simulink model "PID_noise_filter"  (R2020b)
settings: Solver=VariableStepAuto  StartTime=0.0  StopTime=300  RelTol=1e-3
libraries: pid_lib x6, simulink x4, dsparch4 x2
settings Model: Creator=Obsidian  LastModifiedBy=Obsidian

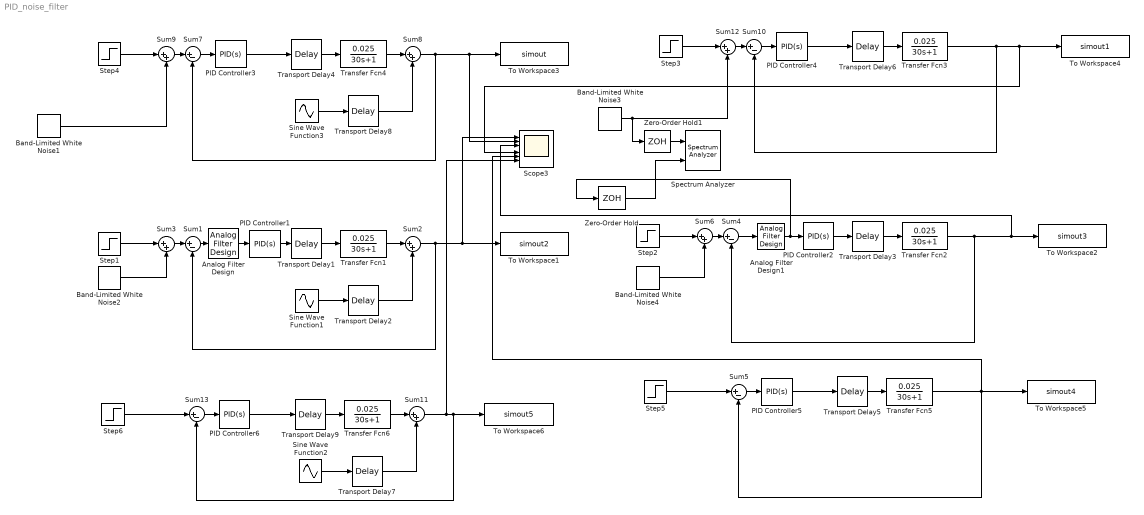
== system PID_noise_filter ==
  Analog Filter Design : dsparch4/Analog Filter Design  method=Butterworth  filttype=Lowpass  N=5  Wlo=62.8  Whi=80  Rp=2  Rs=40
  Analog Filter Design1 : dsparch4/Analog Filter Design  method=Butterworth  filttype=Lowpass  N=5  Wlo=62.8  Whi=80  Rp=2  Rs=40
  Band-Limited White Noise{1..4} (4 alike) : simulink/Sources/Band-Limited White Noise  Cov=[0.1]  Ts=0.01  seed=[23341]
  PID Controller{1..6} (6 alike) : pid_lib/PID Controller  Controller=PID  Form=Parallel  TimeDomain=Continuous-time  UseExternalTs=off  SampleTime=-1  IntegratorMethod=Forward Euler  FilterMethod=Forward Euler  ControllerParametersSource=internal  P=91.1934989789184  I=4.3602787236588  D=159.272174237234  UseFilter=on  N=0.14098946944392  TunerSelectOption=Transfer Function Based (PID Tuner App)  InitialConditionSource=internal  InitialConditionForIntegrator=0  InitialConditionForFilter=0  DifferentiatorICPrevScaledInput=0  ExternalReset=none  TrackingMode=off  Kt=1  LimitOutput=on  SatLimitsSource=internal  UpperSaturationLimit=200  LowerSaturationLimit=0  LinearizeAsGain=on  AntiWindupMode=none  Kb=1  POutMin=[]  POutMax=[]  IOutMin=[]  IOutMax=[]  DOutMin=[]  DOutMax=[]  NOutMin=[]  NOutMax=[]  SumOutMin=[]  SumOutMax=[]  SaturationOutMin=[]  SaturationOutMax=[]  PParamMin=[]  PParamMax=[]  IParamMin=[]  IParamMax=[]  DParamMin=[]  DParamMax=[]  NParamMin=[]  NParamMax=[]  KbParamMin=[]  KbParamMax=[]  KtParamMin=[]  KtParamMax=[]  KbOutMin=[]  KbOutMax=[]  KtOutMin=[]  KtOutMax=[]  IntegratorOutMin=[]  IntegratorOutMax=[]  FilterOutMin=[]  FilterOutMax=[]  SumI1OutMin=[]  SumI1OutMax=[]  SumI2OutMin=[]  SumI2OutMax=[]  SumI3OutMin=[]  SumI3OutMax=[]  SumI4OutMin=[]  SumI4OutMax=[]  SumDOutMin=[]  SumDOutMax=[]  DifferentiatorOutMin=[]  DifferentiatorOutMax=[]  FilterDiffOutCoefMin=[]  FilterDiffOutCoefMax=[]  ReciprocalOutMin=[]  ReciprocalOutMax=[]  SumDenOutMin=[]  SumDenOutMax=[]  SumNumOutMin=[]  SumNumOutMax=[]  DivideOutMin=[]  DivideOutMax=[]  UdiffTsProdOutMin=[]  UdiffTsProdOutMax=[]  NTsProdOutMin=[]  NTsProdOutMax=[]  UintegralTsProdOutMin=[]  UintegralTsProdOutMax=[]  UngainTsProdOutMin=[]  UngainTsProdOutMax=[]  IntegratorContinuousStateAttributes=''  IntegratorStateMustResolveToSignalObject=off  IntegratorRTWStateStorageClass=Auto  FilterContinuousStateAttributes=''  FilterStateMustResolveToSignalObject=off  FilterRTWStateStorageClass=Auto  ParallelPVariant=InternalParameters  IdealPVariant=Disabled  IVariant=InternalParameters  DVariant=InternalParameters  IntegratorVariant=Continuous  SatVariant=Enabled  AWVariant=Passthrough  PCopyVariant=Disabled  TRVariant=Disabled  FdbkBlocksVariant=Forward  IdealPFdbkVariant=Disabled  SatFdbkVariant=Disabled  DerivativeFilterVariant=ContFilter  NVariant=InternalParameters  NCopyVariant=Disabled  FilterICVariant=InternalICsFilter  IntegratorICVariant=InternalICs  ExternalResetVariant=Disabled  TRSumVariant=Passthrough  SumFdbkVariant=Disabled  SumVariant=Sum_PID  TsampFilterVariant=InternalTs  TsampNgainVariant=Passthrough  TsampIntegralVariant=Passthrough  ExternalSaturationOutDataTypeStr=Inherit: Same as second input
  Scope3 : Scope  NumInputPorts=7
  Sine Wave Function1 : Sin  Amplitude=0.03  Frequency=8  SampleTime=0
  Sine Wave Function2 : Sin  Amplitude=0.03  Frequency=8  SampleTime=0
  Sine Wave Function3 : Sin  Amplitude=0.03  Frequency=8  SampleTime=0
  Spectrum Analyzer : SpectrumAnalyzer  NumInputPorts=2
  Step{1..6} (6 alike) : Step  Time=0  After=2  SampleTime=0.01
  Sum{1,4..5,7,10,13} (6 alike) : Sum  Inputs=|+-
  Sum{2..3,6,8..9,11..12} (7 alike) : Sum  Inputs=|++
  To Workspace1 : ToWorkspace  VariableName=simout2  SaveFormat=Structure With Time  SampleTime=-1
  To Workspace2 : ToWorkspace  VariableName=simout3  SaveFormat=Structure With Time  SampleTime=-1
  To Workspace3 : ToWorkspace  VariableName=simout  SaveFormat=Structure With Time  SampleTime=-1
  To Workspace4 : ToWorkspace  VariableName=simout1  SaveFormat=Structure With Time  SampleTime=-1
  To Workspace5 : ToWorkspace  VariableName=simout4  SaveFormat=Structure With Time  SampleTime=-1
  To Workspace6 : ToWorkspace  VariableName=simout5  SaveFormat=Structure With Time  SampleTime=-1
  Transfer Fcn{1..6} (6 alike) : TransferFcn  Numerator=[0.025]  Denominator=[30 1]
  Transport Delay{1..9} (9 alike) : TransportDelay  DelayTime=5
  Zero-Order Hold : ZeroOrderHold  SampleTime=-1
  Zero-Order Hold1 : ZeroOrderHold  SampleTime=-1
  wires:
  Sum8/1 -> Scope3/2, To Workspace3/1, Sum7/2
  Transport Delay4/1 -> Transfer Fcn4/1
  Transfer Fcn4/1 -> Sum8/1
  Sum7/1 -> PID Controller3/1
  PID Controller3/1 -> Transport Delay4/1
  Sine Wave Function3/1 -> Transport Delay8/1
  Sum9/1 -> Sum7/1
  Step4/1 -> Sum9/1
  Sum2/1 -> Scope3/1, To Workspace1/1, Sum1/2
  PID Controller1/1 -> Transport Delay1/1
  Sine Wave Function1/1 -> Transport Delay2/1
  Step1/1 -> Sum3/1
  Transfer Fcn1/1 -> Sum2/1
  Sum3/1 -> Sum1/1
  Transport Delay1/1 -> Transfer Fcn1/1
  Band-Limited White Noise1/1 -> Sum9/2
  Sum6/1 -> Sum4/1
  Step2/1 -> Sum6/1
  Transport Delay3/1 -> Transfer Fcn2/1
  Sum4/1 -> Analog Filter Design1/1
  Transfer Fcn2/1 -> Scope3/3, To Workspace2/1, Sum4/2
  PID Controller2/1 -> Transport Delay3/1
  Band-Limited White Noise3/1 -> Zero-Order Hold1/1, Sum12/2
  Transfer Fcn3/1 -> Scope3/5, To Workspace4/1, Sum10/2
  Sum10/1 -> PID Controller4/1
  PID Controller4/1 -> Transport Delay6/1
  Step3/1 -> Sum12/1
  Sum12/1 -> Sum10/1
  Transport Delay6/1 -> Transfer Fcn3/1
  Zero-Order Hold/1 -> Spectrum Analyzer/2
  Zero-Order Hold1/1 -> Spectrum Analyzer/1
  Transport Delay2/1 -> Sum2/2
  Transport Delay8/1 -> Sum8/2
  Analog Filter Design1/1 -> Zero-Order Hold/1, PID Controller2/1
  Band-Limited White Noise4/1 -> Sum6/2
  Sum1/1 -> Analog Filter Design/1
  Analog Filter Design/1 -> PID Controller1/1
  Band-Limited White Noise2/1 -> Sum3/2
  Transfer Fcn5/1 -> To Workspace5/1, Scope3/6, Sum5/2
  Sum5/1 -> PID Controller5/1
  PID Controller5/1 -> Transport Delay5/1
  Transport Delay5/1 -> Transfer Fcn5/1
  Step5/1 -> Sum5/1
  Transport Delay7/1 -> Sum11/2
  Sine Wave Function2/1 -> Transport Delay7/1
  PID Controller6/1 -> Transport Delay9/1
  Sum13/1 -> PID Controller6/1
  Step6/1 -> Sum13/1
  Transfer Fcn6/1 -> Sum11/1
  Transport Delay9/1 -> Transfer Fcn6/1
  Sum11/1 -> Scope3/7, Sum13/2, To Workspace6/1
